simulink model "Modele_pendule_d"  (R2020b)
settings: Solver=VariableStepAuto  StartTime=0.0  StopTime=100  RelTol=1e-3
undefined symbols (not defined in the file or in its folder): kd, ki, kp, Kx, now, x_0
libraries: pid_lib x1
settings Model: Creator=georgesghazi  LastModifiedBy=georgesghazi

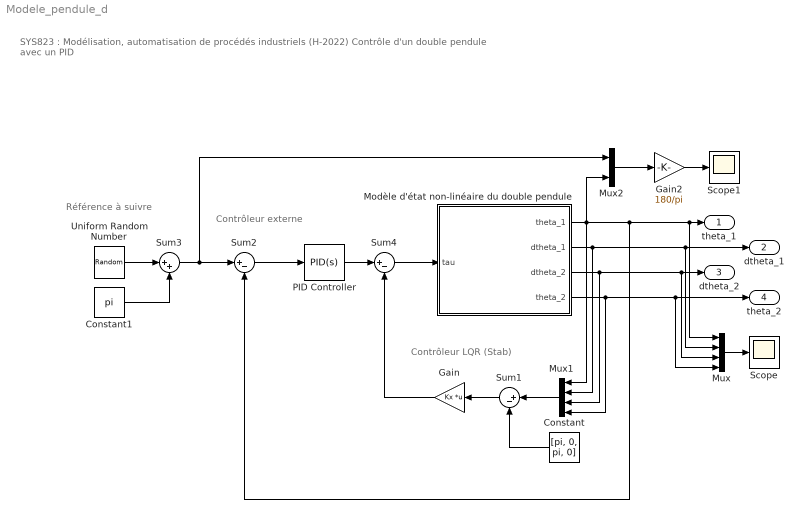
== system Modele_pendule_d ==
  note: Contrôleur externe
  note: Référence à suivre
  note: Contrôleur LQR (Stab)
  note: SYS823 : Modélisation, automatisation de procédés industriels (H-2022)
      |
      | Contrôle d'un double pendule avec un PID
  Constant : Constant  Value=[pi, 0, pi, 0]
  Constant1 : Constant  Value=pi
  Gain : Gain  Gain=Kx  Multiplication=Matrix(K*u) (u vector)
  Gain2 : Gain  Gain=180/pi
  Modèle d'état non-linéaire du double pendule : Subsystem
  Mux : Mux
  Mux1 : Mux
  Mux2 : Mux  Inputs=2
  PID Controller : pid_lib/PID Controller  Controller=PID  Form=Parallel  TimeDomain=Continuous-time  UseExternalTs=off  SampleTime=-1  IntegratorMethod=Forward Euler  FilterMethod=Forward Euler  ControllerParametersSource=internal  P=kp  I=ki  D=kd  UseFilter=on  N=100000  TunerSelectOption=Transfer Function Based (PID Tuner App)  InitialConditionSource=internal  InitialConditionForIntegrator=0  InitialConditionForFilter=0  DifferentiatorICPrevScaledInput=0  ExternalReset=none  TrackingMode=off  Kt=1  LimitOutput=off  SatLimitsSource=internal  UpperSaturationLimit=inf  LowerSaturationLimit=-inf  LinearizeAsGain=on  AntiWindupMode=none  Kb=1  POutMin=[]  POutMax=[]  IOutMin=[]  IOutMax=[]  DOutMin=[]  DOutMax=[]  NOutMin=[]  NOutMax=[]  SumOutMin=[]  SumOutMax=[]  SaturationOutMin=[]  SaturationOutMax=[]  PParamMin=[]  PParamMax=[]  IParamMin=[]  IParamMax=[]  DParamMin=[]  DParamMax=[]  NParamMin=[]  NParamMax=[]  KbParamMin=[]  KbParamMax=[]  KtParamMin=[]  KtParamMax=[]  KbOutMin=[]  KbOutMax=[]  KtOutMin=[]  KtOutMax=[]  IntegratorOutMin=[]  IntegratorOutMax=[]  FilterOutMin=[]  FilterOutMax=[]  SumI1OutMin=[]  SumI1OutMax=[]  SumI2OutMin=[]  SumI2OutMax=[]  SumI3OutMin=[]  SumI3OutMax=[]  SumI4OutMin=[]  SumI4OutMax=[]  SumDOutMin=[]  SumDOutMax=[]  DifferentiatorOutMin=[]  DifferentiatorOutMax=[]  FilterDiffOutCoefMin=[]  FilterDiffOutCoefMax=[]  ReciprocalOutMin=[]  ReciprocalOutMax=[]  SumDenOutMin=[]  SumDenOutMax=[]  SumNumOutMin=[]  SumNumOutMax=[]  DivideOutMin=[]  DivideOutMax=[]  UdiffTsProdOutMin=[]  UdiffTsProdOutMax=[]  NTsProdOutMin=[]  NTsProdOutMax=[]  UintegralTsProdOutMin=[]  UintegralTsProdOutMax=[]  UngainTsProdOutMin=[]  UngainTsProdOutMax=[]  IntegratorContinuousStateAttributes=''  IntegratorStateMustResolveToSignalObject=off  IntegratorRTWStateStorageClass=Auto  FilterContinuousStateAttributes=''  FilterStateMustResolveToSignalObject=off  FilterRTWStateStorageClass=Auto  ParallelPVariant=InternalParameters  IdealPVariant=Disabled  IVariant=InternalParameters  DVariant=InternalParameters  IntegratorVariant=Continuous  SatVariant=Disabled  AWVariant=Passthrough  PCopyVariant=Disabled  TRVariant=Disabled  FdbkBlocksVariant=Forward  IdealPFdbkVariant=Disabled  SatFdbkVariant=Disabled  DerivativeFilterVariant=ContFilter  NVariant=InternalParameters  NCopyVariant=Disabled  FilterICVariant=InternalICsFilter  IntegratorICVariant=InternalICs  ExternalResetVariant=Disabled  TRSumVariant=Passthrough  SumFdbkVariant=Disabled  SumVariant=Sum_PID  TsampFilterVariant=InternalTs  TsampNgainVariant=Passthrough  TsampIntegralVariant=Passthrough  ExternalSaturationOutDataTypeStr=Inherit: Same as second input
  Scope : Scope
  Scope1 : Scope
  Sum1 : Sum  Inputs=|+-
  Sum2 : Sum  Inputs=|+-
  Sum3 : Sum  Inputs=|++
  Sum4 : Sum  Inputs=|+-
  Uniform Random Number : UniformRandomNumber  Minimum=-25*pi/180  Maximum=+25*pi/180  Seed=round(now)  SampleTime=20
  theta_1 : Outport
  dtheta_1 : Outport  Port=2
  dtheta_2 : Outport  Port=3
  theta_2 : Outport  Port=4
  wires:
  Mux/1 -> Scope/1
  Modèle d'état non-linéaire du double pendule/1(theta_1) -> Mux/1, theta_1/1, Sum2/2, Mux2/2, Mux1/1
  Modèle d'état non-linéaire du double pendule/2(dtheta_1) -> Mux1/2, Mux/2, dtheta_1/1
  Modèle d'état non-linéaire du double pendule/3(dtheta_2) -> Mux1/3, Mux/3, dtheta_2/1
  Modèle d'état non-linéaire du double pendule/4(theta_2) -> Mux1/4, theta_2/1, Mux/4
  Sum4/1 -> Modèle d'état non-linéaire du double pendule/1(tau)
  Sum1/1 -> Gain/1
  Mux1/1 -> Sum1/1
  Constant/1 -> Sum1/2
  Sum2/1 -> PID Controller/1
  Sum3/1 -> Sum2/1, Mux2/1
  Gain/1 -> Sum4/2
  Uniform Random Number/1 -> Sum3/1
  Constant1/1 -> Sum3/2
  Mux2/1 -> Gain2/1
  Gain2/1 -> Scope1/1
  PID Controller/1 -> Sum4/1

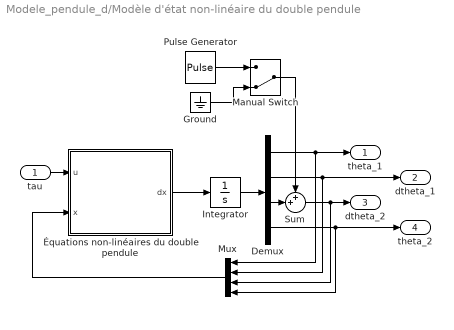
== system Modele_pendule_d/Modèle d'état non-linéaire du double pendule ==
  tau : Inport
  Demux : Demux
  Ground : Ground
  Integrator : Integrator  InitialCondition=x_0
  Manual Switch : ManualSwitch  CurrentSetting=0
  Mux : Mux
  Pulse Generator : DiscretePulseGenerator  PulseType=Time based  Amplitude=5*pi/180  Period=10
  Sum : Sum  Inputs=++|
  Équations non-linéaires du double pendule : MATLAB Function  TreatAsAtomicUnit=on
  theta_1 : Outport
  dtheta_1 : Outport  Port=2
  dtheta_2 : Outport  Port=3
  theta_2 : Outport  Port=4
  wires:
  Équations non-linéaires du double pendule/1(dx) -> Integrator/1
  Integrator/1 -> Demux/1
  tau/1 -> Équations non-linéaires du double pendule/1(u)
  Demux/2 -> Mux/2, dtheta_1/1
  Demux/4 -> Mux/4, theta_2/1
  Demux/1 -> theta_1/1, Mux/1
  Mux/1 -> Équations non-linéaires du double pendule/2(x)
  Demux/3 -> Sum/2
  Sum/1 -> Mux/3, dtheta_2/1
  Pulse Generator/1 -> Manual Switch/1
  Ground/1 -> Manual Switch/2
  Manual Switch/1 -> Sum/1

== matlab function Modele_pendule_d/Modèle d'état non-linéaire du double pendule/Équations non-linéaires du double pendule ==
  data: u input; dx output; x input
function dx = fcn(u, x)
% Déclaration des constantes 
m_1 = 1; m_2 = 1;
l_1 = 2; l_2 = 2;
g_0 = 9.81;

% Calcul de la dérivée du vecteur d'état
dx = zeros(size(x));

dx(1) = x(2);
dx(2) = -(l_1*l_2*m_2*sin(x(1) - x(3))*x(4)^2 - u - l_1*m_2*cos(x(1) - x(3))*(g_0*sin(x(3)) - ...
    l_1*x(2)^2*sin(x(1) - x(3))) + g_0*l_1*m_1*sin(x(1)) + g_0*l_1*m_2*sin(x(1)))/(l_1^2*m_1 + l_1^2*m_2);
dx(3) = x(4);
dx(4) = (l_1*sin(x(1) - x(3))*x(2)^2 - g_0*sin(x(3)) + (l_1*cos(x(1) - x(3))*...
    (l_1*l_2*m_2*sin(x(1) - x(3))*x(4)^2 - u + g_0*l_1*m_1*sin(x(1)) + ...
    g_0*l_1*m_2*sin(x(1))))/(l_1^2*m_1 + l_1^2*m_2))/l_2;
